simulink library "lib_Convection_TurbFlatPlate"  (R2015a)
settings: Solver=ode45  StartTime=0.0  StopTime=10.0  RelTol=1e-3
libraries: simulink x4
settings Model: Creator=jlkratz  LastModifiedBy=jlkratz

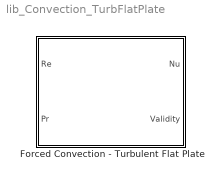
== system lib_Convection_TurbFlatPlate ==
  Forced Convection - Turbulent Flat Plate : Subsystem  mask(TSAT: Turbulent Flat Plate){LocalOrAvg_M=Local Nusselt number, IsothermOrIsoflux_M=Isothermal Plate}
      mask help:
      | This block estimates the Nusselt number of a turbulent external flow over an isothermal or isoflux flat plate. It can either calculate the local or average Nusselt number over 1 surface of the plate. If the average Nusselt number is to be calcualted then assure the charateristic length used to calculate the Reynolds Number is the full length of the plate. Note that all fluid properrties should be evaluated at film temperature (average of the bulk fluid and surface temperatures). Beyond the flow being turbulent the implemented correlations also requires:
      |
      | 500000 <= Re <= 10^8
      | 0.6 <= Pr <= 60
      |
      | If all of these contraint are not met then the "Validity" output will be 1, and otherwise will be 0. For more information on the implemented correlations and function of the block, see the block help menu.
      mask Help: web(which('Convection_TSAT_TurbulentFlatPlate.html'),'-helpbrowser')
      mask TypeOptions LocalOrAvg_M: Local Nusselt number | Average Nusselt number
      mask TypeOptions IsothermOrIsoflux_M: Isothermal Plate | Isoflux Plate

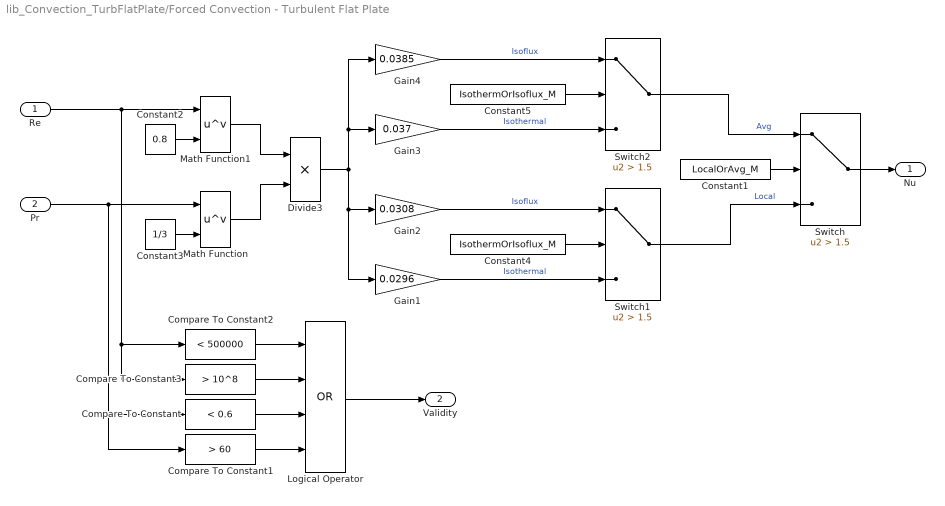
== system lib_Convection_TurbFlatPlate/Forced Convection - Turbulent Flat Plate ==
  Re : Inport
  Pr : Inport  Port=2
  Compare To Constant : simulink/Logic and Bit Operations/Compare To Constant  relop=<  const=0.6  OutDataTypeStr=boolean
  Compare To Constant1 : simulink/Logic and Bit Operations/Compare To Constant  relop=>  const=60  OutDataTypeStr=boolean
  Compare To Constant2 : simulink/Logic and Bit Operations/Compare To Constant  relop=<  const=500000  OutDataTypeStr=boolean
  Compare To Constant3 : simulink/Logic and Bit Operations/Compare To Constant  relop=>  const=10^8  OutDataTypeStr=boolean
  Constant1 : Constant  Value=LocalOrAvg_M
  Constant2 : Constant  Value=0.8
  Constant3 : Constant  Value=1/3
  Constant4 : Constant  Value=IsothermOrIsoflux_M
  Constant5 : Constant  Value=IsothermOrIsoflux_M
  Divide3 : Product  Inputs=**
  Gain1 : Gain  Gain=0.0296
  Gain2 : Gain  Gain=0.0308
  Gain3 : Gain  Gain=0.037
  Gain4 : Gain  Gain=0.0385
  Logical Operator : Logic  Operator=OR  Inputs=4  AllPortsSameDT=off  OutDataTypeStr=boolean
  Math Function : Math  Operator=pow  SaturateOnIntegerOverflow=on
  Math Function1 : Math  Operator=pow  SaturateOnIntegerOverflow=on
  Switch : Switch  Criteria=u2 > Threshold  Threshold=1.5
  Switch1 : Switch  Criteria=u2 > Threshold  Threshold=1.5
  Switch2 : Switch  Criteria=u2 > Threshold  Threshold=1.5
  Nu : Outport
  Validity : Outport  Port=2
  wires:
  Gain4/1 -> Switch2/1  "Isoflux"
  Gain3/1 -> Switch2/3  "Isothermal"
  Constant5/1 -> Switch2/2
  Gain1/1 -> Switch1/3  "Isothermal"
  Gain2/1 -> Switch1/1  "Isoflux"
  Constant4/1 -> Switch1/2
  Logical Operator/1 -> Validity/1
  Compare To Constant1/1 -> Logical Operator/4
  Compare To Constant/1 -> Logical Operator/3
  Compare To Constant3/1 -> Logical Operator/2
  Compare To Constant2/1 -> Logical Operator/1
  Switch1/1 -> Switch/3  "Local"
  Switch2/1 -> Switch/1  "Avg"
  Constant1/1 -> Switch/2
  Divide3/1 -> Gain3/1, Gain4/1, Gain1/1, Gain2/1
  Math Function/1 -> Divide3/2
  Math Function1/1 -> Divide3/1
  Constant2/1 -> Math Function1/2
  Switch/1 -> Nu/1
  Constant3/1 -> Math Function/2
  Pr/1 -> Compare To Constant/1, Compare To Constant1/1, Math Function/1
  Re/1 -> Math Function1/1, Compare To Constant3/1, Compare To Constant2/1
